simulink model "U2_asim"  (R2022b)
settings: Solver=ode4  StartTime=0.0  StopTime=10.0  FixedStep=tstep  RelTol=1e-3
undefined symbols (not defined in the file): den, num
settings Model: Creator=dipte  LastModifiedBy=dipte
settings DataIOCC: ReturnWorkspaceOutputs=off

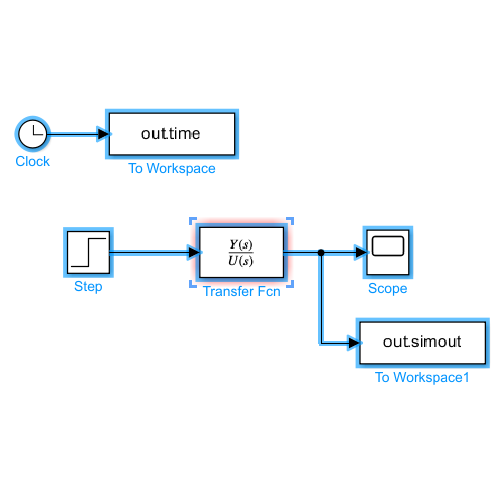
[thumbnail: Simulink's stored preview of the top-level diagram]
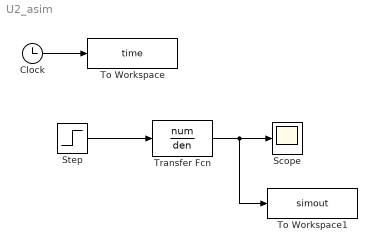
== system U2_asim ==
  Clock : Clock
  Scope : Scope
  Step : Step  Time=0  SampleTime=0
  To Workspace : ToWorkspace  VariableName=time  SampleTime=-1
      settings: Save2DSignal=2-D array (concatenate along first dimension)
  To Workspace1 : ToWorkspace  VariableName=simout  SampleTime=-1
      settings: Save2DSignal=2-D array (concatenate along first dimension)
  Transfer Fcn : TransferFcn  Numerator=num  Denominator=den
  wires:
  Transfer Fcn/1 -> To Workspace1/1, Scope/1
  Clock/1 -> To Workspace/1
  Step/1 -> Transfer Fcn/1
